simulink model "Load_Transfer"  (R2020a)
settings: Solver=VariableStepAuto  StartTime=0.0  StopTime=10.0  RelTol=1e-3
values from neighbouring files (symbols this model uses):
  ARB_arm : value not decoded    [Properties.sldd]
  ARB_torsional_rigidity = 1.0    [Properties.sldd]
  Car_mass = 245.0    [Properties.sldd]
  CG_x = 0.6    [Properties.sldd]
  CG_z = 0.3    [Properties.sldd]
  Shock_damping : value not decoded    [Properties.sldd]
  Shock_stiffness : value not decoded    [Properties.sldd]
  Track_width = 2.0    [Properties.sldd]
  Wheelbase = 1.2    [Properties.sldd]
settings Model: DataDictionary=Properties.sldd  Creator=Matthew  LastModifiedBy=Matthew
settings ModelReferenceCC: ModelReferenceMinAlgLoopOccurrences=on

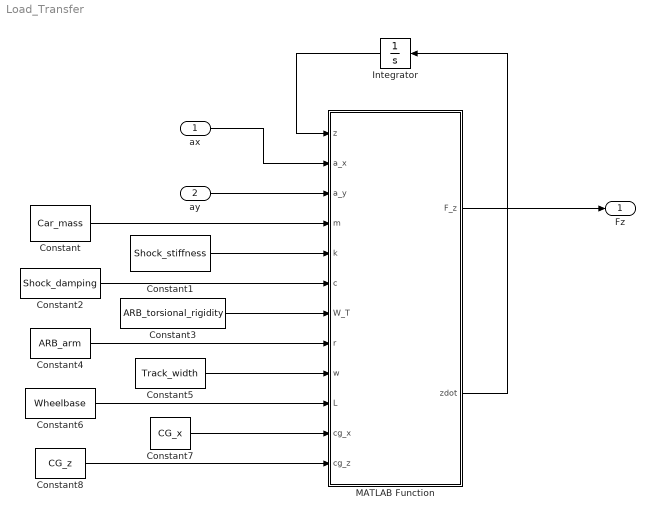
== system Load_Transfer ==
  ax : Inport
  ay : Inport  Port=2
  Constant : Constant  Value=Car_mass
  Constant1 : Constant  Value=Shock_stiffness
  Constant2 : Constant  Value=Shock_damping
  Constant3 : Constant  Value=ARB_torsional_rigidity
  Constant4 : Constant  Value=ARB_arm
  Constant5 : Constant  Value=Track_width
  Constant6 : Constant  Value=Wheelbase
  Constant7 : Constant  Value=CG_x
  Constant8 : Constant  Value=CG_z
  Integrator : Integrator  InitialCondition=[0,0,0,0]
  MATLAB Function : MATLAB Function
  Fz : Outport
  wires:
  MATLAB Function/2(zdot) -> Integrator/1
  Integrator/1 -> MATLAB Function/1(z)
  ax/1 -> MATLAB Function/2(a_x)
  MATLAB Function/1(F_z) -> Fz/1
  ay/1 -> MATLAB Function/3(a_y)
  Constant/1 -> MATLAB Function/4(m)
  Constant1/1 -> MATLAB Function/5(k)
  Constant2/1 -> MATLAB Function/6(c)
  Constant3/1 -> MATLAB Function/7(W_T)
  Constant4/1 -> MATLAB Function/8(r)
  Constant5/1 -> MATLAB Function/9(w)
  Constant6/1 -> MATLAB Function/10(L)
  Constant7/1 -> MATLAB Function/11(cg_x)
  Constant8/1 -> MATLAB Function/12(cg_z)

== matlab function Load_Transfer/MATLAB Function ==
  data: z input; F_z output; a_x input; a_y input; m input; k input; c input; W_T input; r input; w input; L input; zdot output; cg_x input; cg_z input
function [F_z,zdot] = normal_forces(z,a_x,a_y,m,k,c,W_T,r,w,L, cg_x,cg_z)
g=9.81;
A=[
    0       0       0       0       L       L       0       0;
    0       0       0       0       w       0       w       0;
    0       0       0       0       1       1       1       1;
    c(1)    0       0       0       1       0       0       0;
    0       c(1)    0       0       0       1       0       0;
    0       0       c(2)    0       0       0       1       0;
    0       0       0       c(2)    0       0       0       1;
    1       -1      -1      1       0       0       0       0;
    ];
b=[
    -m*g*cg_x+a_x*m*cg_z;
    -m*g*w/2+a_y*m*cg_z;
    -m*g;
    -(k(1)+W_T/(w*r(1)^2))*z(1)+W_T/(w*r(1)^2)*z(2);
    -(k(1)+W_T/(w*r(1)^2))*z(2)+W_T/(w*r(1)^2)*z(1);
    -(k(2)+W_T/(w*r(2)^2))*z(3)+W_T/(w*r(2)^2)*z(4);
    -(k(2)+W_T/(w*r(2)^2))*z(4)+W_T/(w*r(2)^2)*z(3);
    0
    ];

x=A\b;
zdot=x(1:4,1);
F_z=x(5:8,1);
